simulink model "LIMITATIONS"  (R2024b)
settings: Solver=FixedStepAuto  StartTime=0.0  StopTime=10.0  RelTol=1e-3  EnableMultiTasking=on
settings Model: DataDictionary=Master_Dictionary.sldd  EnableAccessToBaseWorkspace=off  Creator=torni  LastModifiedBy=Will
settings OptimizationCC: DefaultParameterBehavior=Inlined  EnhancedBackFolding=on  PassReuseOutputArgsAs=Individual arguments  ZeroExternalMemoryAtStartup=off  ZeroInternalMemoryAtStartup=off  MaxStackSize=8192  OptimizeBlockOrder=speed  DifferentSizesBufferReuse=on  OptimizationCustomize=off  EfficientTunableParamExpr=on
settings DebuggingCC: ParameterTunabilityLossMsg=error
settings HardwareCC: ProdBitPerPointer=32  ProdBitPerSizeT=32  ProdBitPerPtrDiffT=32  ProdLargestAtomicInteger=Long  ProdLargestAtomicFloat=Double  ProdWordSize=32  ProdLongLongMode=on  ProdHWDeviceType=ARM Compatible->ARM Cortex-M
settings SFSimCC: MATLABDynamicMemAlloc=off
settings RTWCC: Description=Embedded Coder  SystemTargetFile=ert.tlc  HardwareBoard=STM32H7xx Based (Single-core)  TemplateMakefile=ert_default_tmf  Toolchain=GNU Tools for ARM Embedded Processors
settings CodeAppCC: ForceParamTrailComments=on  IgnoreCustomStorageClasses=off  OperatorAnnotations=on  SimulinkDataObjDesc=on  SFDataObjDesc=on  InsertBlockDesc=on
settings ERTTargetCC: TargetLangStandard=C99 (ISO)  CodeReplacementLibrary=ARM Cortex-M  ExtModeTransport=3  ExtModeStaticAlloc=on  ExtModeStaticAllocSize=2048  ExtModeMexFile=ext_xcp  ExtModeIntrfLevel=Level2 - Open

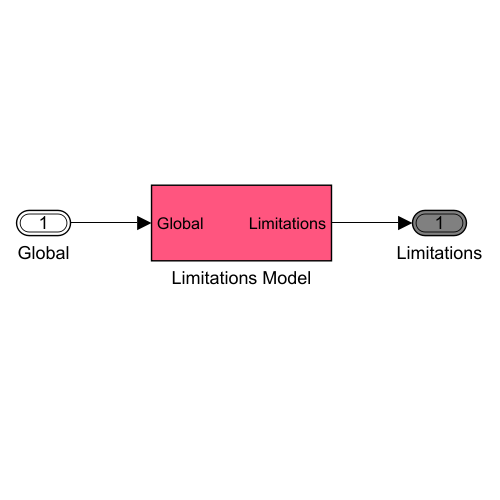
[thumbnail: Simulink's stored preview of the top-level diagram]
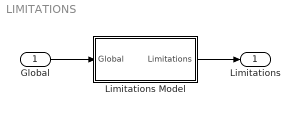
== system LIMITATIONS ==
  "Global " : Inport  OutDataTypeStr=Bus: Global
  "Limitations Model " : Subsystem
  Limitations : Outport  OutDataTypeStr=Bus: Limitations  VectorParamsAs1DForOutWhenUnconnected=off
  wires:
  "Global "/1 -> "Limitations Model "/1(Global)
  "Limitations Model "/1(Limitations) -> Limitations/1

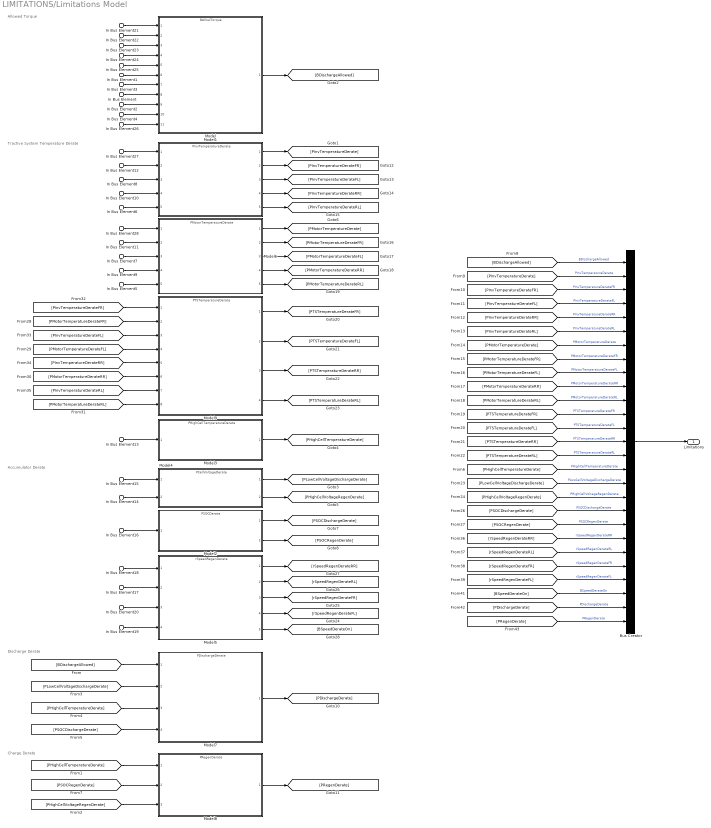
== system LIMITATIONS/Limitations Model  ==
  note: Allowed Torque
  note: Discharge Derate
  note: Charge Derate
  note: Tractive System Temperature Derate
  note: Accumulator Derate
  In Bus Element : Inport  PortName=Global  Element=InverterSignals.InverterRLSignals.nMotorRL
  In Bus Element5 : Inport  PortName=Global  Element=InverterSignals.InverterRLSignals.TMotorRL
  In Bus Element6 : Inport  PortName=Global  Element=InverterSignals.InverterRLSignals.TInvRL
  In Bus Element1 : Inport  PortName=Global  Element=InverterSignals.InverterFLSignals.nMotorFL
  In Bus Element7 : Inport  PortName=Global  Element=InverterSignals.InverterFLSignals.TMotorFL
  In Bus Element8 : Inport  PortName=Global  Element=InverterSignals.InverterFLSignals.TInvFL
  In Bus Element2 : Inport  PortName=Global  Element=InverterSignals.InverterRRSignals.nMotorRR
  In Bus Element9 : Inport  PortName=Global  Element=InverterSignals.InverterRRSignals.TMotorRR
  In Bus Element10 : Inport  PortName=Global  Element=InverterSignals.InverterRRSignals.TInvRR
  In Bus Element3 : Inport  PortName=Global  Element=InverterSignals.InverterFRSignals.nMotorFR
  In Bus Element11 : Inport  PortName=Global  Element=InverterSignals.InverterFRSignals.TMotorFR
  In Bus Element12 : Inport  PortName=Global  Element=InverterSignals.InverterFRSignals.TInvFR
  In Bus Element4 : Inport  PortName=Global  Element=BMSSignals.IIVTS
  In Bus Element13 : Inport  PortName=Global  Element=BMSSignals.TCellMax
  In Bus Element14 : Inport  PortName=Global  Element=BMSSignals.VCellMax
  In Bus Element15 : Inport  PortName=Global  Element=BMSSignals.VCellMin
  In Bus Element16 : Inport  PortName=Global  Element=BMSSignals.VDCAccumulator
  In Bus Element17 : Inport  PortName=Global  Element=WheelSpeeds.vWheelRL
  In Bus Element18 : Inport  PortName=Global  Element=WheelSpeeds.vWheelRR
  In Bus Element19 : Inport  PortName=Global  Element=WheelSpeeds.vWheelFL
  In Bus Element20 : Inport  PortName=Global  Element=WheelSpeeds.vWheelFR
  In Bus Element21 : Inport  PortName=Global  Element=Stateflow.BReadyToDrive
  In Bus Element22 : Inport  PortName=Global  Element=Systems.BBrakeOn
  In Bus Element23 : Inport  PortName=Global  Element=Systems.BThrottleError
  In Bus Element24 : Inport  PortName=Global  Element=Systems.BBrakeError
  In Bus Element25 : Inport  PortName=Global  Element=Systems.BAppsOK
  In Bus Element26 : Inport  PortName=Global  Element=Systems.BRegenOn
  In Bus Element27 : Inport  PortName=Global  Element=Systems.TInvMax
  In Bus Element28 : Inport  PortName=Global  Element=Systems.TMotorMax
  Bus Creator : BusCreator  Inputs=27  OutDataTypeStr=Bus: Limitations
  Model : ModelReference  ModelNameDialog=BAllowTorque  SimulationMode=Normal  ModelReferenceVersion=13.6
  Model1 : ModelReference  ModelNameDialog=PInvTemperatureDerate.slx  SimulationMode=Normal  ModelReferenceVersion=13.6
  Model2 : ModelReference  ModelNameDialog=PSOCDerate.slx  SimulationMode=Normal  ModelReferenceVersion=13.6
  Model3 : ModelReference  ModelNameDialog=PHighCellTemperatureDerate.slx  SimulationMode=Normal  ModelReferenceVersion=13.6
  Model4 : ModelReference  ModelNameDialog=PCellVoltageDerate.slx  SimulationMode=Normal  ModelReferenceVersion=13.6
  Model5 : ModelReference  ModelNameDialog=rSpeedRegenDerate.slx  SimulationMode=Normal  ModelReferenceVersion=13.6
  Model6 : ModelReference  ModelNameDialog=PMotorTemperatureDerate.slx  SimulationMode=Normal  ModelReferenceVersion=13.6
  Model7 : ModelReference  ModelNameDialog=PDischargeDerate.slx  SimulationMode=Normal  ModelReferenceVersion=13.6
  Model8 : ModelReference  ModelNameDialog=PRegenDerate.slx  SimulationMode=Normal  ModelReferenceVersion=13.6
  Model9 : ModelReference  ModelNameDialog=PTSTemperatureDerate.slx  SimulationMode=Normal  ModelReferenceVersion=13.6
  Limitations : Outport  OutDataTypeStr=Bus: Limitations  VectorParamsAs1DForOutWhenUnconnected=off  LockScale=on
  wires:
  Model/1 -> [BDischargeAllowed]
  In Bus Element27/1 -> Model1/1
  Model1/1 -> [PInvTemperatureDerate]
  Bus Creator/1 -> Limitations/1
  In Bus Element15/1 -> Model4/1
  Model4/1 -> [PLowCellVoltageDischargeDerate]
  In Bus Element13/1 -> Model3/1
  Model3/1 -> [PHighCellTemperatureDerate]
  In Bus Element28/1 -> Model6/1
  Model6/1 -> [PMotorTemperatureDerate]
  In Bus Element16/1 -> Model2/1
  Model2/1 -> [PSOCDischargeDerate]
  Model2/2 -> [PSOCRegenDerate]
  Model5/1 -> [rSpeedRegenDerateRR]
  [PSOCDischargeDerate] -> Model7/4
  [PHighCellTemperatureDerate] -> Model7/3
  Model7/1 -> [PDischargeDerate]
  [PSOCRegenDerate] -> Model8/2
  Model8/1 -> [PRegenDerate]
  [BDischargeAllowed] -> Model7/1
  Model1/2 -> [PInvTemperatureDerateFR]
  Model1/3 -> [PInvTemperatureDerateFL]
  Model1/4 -> [PInvTemperatureDerateRR]
  Model1/5 -> [PInvTemperatureDerateRL]
  In Bus Element12/1 -> Model1/2
  In Bus Element8/1 -> Model1/3
  In Bus Element10/1 -> Model1/4
  In Bus Element6/1 -> Model1/5
  Model6/2 -> [PMotorTemperatureDerateFR]
  Model6/3 -> [PMotorTemperatureDerateFL]
  Model6/4 -> [PMotorTemperatureDerateRR]
  Model6/5 -> [PMotorTemperatureDerateRL]
  In Bus Element7/1 -> Model6/3
  In Bus Element9/1 -> Model6/4
  In Bus Element5/1 -> Model6/5
  In Bus Element11/1 -> Model6/2
  Model9/1 -> [PTSTemperatureDerateFR]
  Model9/2 -> [PTSTemperatureDerateFL]
  Model9/3 -> [PTSTemperatureDerateRR]
  Model9/4 -> [PTSTemperatureDerateRL]
  [PInvTemperatureDerateRR] -> Model9/5
  [PMotorTemperatureDerateRR] -> Model9/6
  [PInvTemperatureDerateRL] -> Model9/7
  [PMotorTemperatureDerateRL] -> Model9/8
  [PInvTemperatureDerateFL] -> Model9/3
  [PInvTemperatureDerateFR] -> Model9/1
  [PMotorTemperatureDerateFR] -> Model9/2
  [PMotorTemperatureDerateFL] -> Model9/4
  Model5/4 -> [rSpeedRegenDerateFL]
  Model5/3 -> [rSpeedRegenDerateFR]
  Model5/2 -> [rSpeedRegenDerateRL]
  Model5/5 -> [BSpeedDerateOn]
  In Bus Element17/1 -> Model5/2
  In Bus Element18/1 -> Model5/1
  In Bus Element19/1 -> Model5/4
  In Bus Element20/1 -> Model5/3
  [BDischargeAllowed] -> Bus Creator/1  "BDischargeAllowed"
  [PInvTemperatureDerate] -> Bus Creator/2  "PInvTemperatureDerate"
  [PInvTemperatureDerateFR] -> Bus Creator/3  "PInvTemperatureDerateFR"
  [PInvTemperatureDerateFL] -> Bus Creator/4  "PInvTemperatureDerateFL"
  [PInvTemperatureDerateRR] -> Bus Creator/5  "PInvTemperatureDerateRR"
  [PInvTemperatureDerateRL] -> Bus Creator/6  "PInvTemperatureDerateRL"
  [PMotorTemperatureDerateFR] -> Bus Creator/8  "PMotorTemperatureDerateFR"
  [PMotorTemperatureDerate] -> Bus Creator/7  "PMotorTemperatureDerate"
  [PMotorTemperatureDerateFL] -> Bus Creator/9  "PMotorTemperatureDerateFL"
  [PMotorTemperatureDerateRR] -> Bus Creator/10  "PMotorTemperatureDerateRR"
  [PMotorTemperatureDerateRL] -> Bus Creator/11  "PMotorTemperatureDerateRL"
  [PTSTemperatureDerateFR] -> Bus Creator/12  "PTSTemperatureDerateFR"
  [PTSTemperatureDerateFL] -> Bus Creator/13  "PTSTemperatureDerateFL"
  [PTSTemperatureDerateRR] -> Bus Creator/14  "PTSTemperatureDerateRR"
  [PTSTemperatureDerateRL] -> Bus Creator/15  "PTSTemperatureDerateRL"
  [PHighCellTemperatureDerate] -> Bus Creator/16  "PHighCellTemperatureDerate"
  [PLowCellVoltageDischargeDerate] -> Bus Creator/17  "PLowCellVoltageDischargeDerate"
  [PHighCellVoltageRegenDerate] -> Bus Creator/18  "PHighCellVoltageRegenDerate"
  [PSOCDischargeDerate] -> Bus Creator/19  "PSOCDischargeDerate"
  [PSOCRegenDerate] -> Bus Creator/20  "PSOCRegenDerate"
  [rSpeedRegenDerateRR] -> Bus Creator/21  "rSpeedRegenDerateRR"
  [rSpeedRegenDerateRL] -> Bus Creator/22  "rSpeedRegenDerateRL"
  [rSpeedRegenDerateFR] -> Bus Creator/23  "rSpeedRegenDerateFR"
  [rSpeedRegenDerateFL] -> Bus Creator/24  "rSpeedRegenDerateFL"
  [BSpeedDerateOn] -> Bus Creator/25  "BSpeedDerateOn"
  [PDischargeDerate] -> Bus Creator/26  "PDischargeDerate"
  [PRegenDerate] -> Bus Creator/27  "PRegenDerate"
  [PLowCellVoltageDischargeDerate] -> Model7/2
  Model4/2 -> [PHighCellVoltageRegenDerate]
  [PHighCellTemperatureDerate] -> Model8/1
  [PHighCellVoltageRegenDerate] -> Model8/3
  In Bus Element4/1 -> Model/10
  In Bus Element3/1 -> Model/7
  In Bus Element/1 -> Model/8
  In Bus Element1/1 -> Model/6
  In Bus Element2/1 -> Model/9
  In Bus Element14/1 -> Model4/2
  In Bus Element21/1 -> Model/1
  In Bus Element22/1 -> Model/2
  In Bus Element23/1 -> Model/3
  In Bus Element24/1 -> Model/4
  In Bus Element25/1 -> Model/5
  In Bus Element26/1 -> Model/11
